simulink model "simulator_lqr_lpv"  (R2024a)
settings: Solver=FixedStepAuto  StartTime=0.0  StopTime=10  FixedStep=0.01  RelTol=1e-3
values from neighbouring files (symbols this model uses):
  ad = sys_d.A    [Project.m]
  bd = sys_d.B    [Project.m]
  BT_D = Ts * B_T    [Project.m]
  C_T = diag([1, 1, 1])    [Project.m]
  D_T = [0;0;0]    [Project.m]
  K1 = Y1*inv(P)    [Project.m]
  K2 = Y2*inv(P)    [Project.m]
  K3 = Y3*inv(P)    [Project.m]
  K4 = Y4*inv(P)    [Project.m]
  K_lqr = dlqr(ad, bd, Q_lqr, R_lqr)    [Project.m]
  Kk1 = Y1*inv(P)    [Project.m]
  Kk2 = Y2*inv(P)    [Project.m]
  Kk3 = Y3*inv(P)    [Project.m]
  rho1max = maxval    (= 20)    [Project.m]
  rho1min = minval    (= 5)    [Project.m]
  rho2max = 1/minval    (= 0.2)    [Project.m]
  rho2min = 1/maxval    (= 0.05)    [Project.m]
  Ts = 0.01    [Project.m]
  vx = 20    [Project.m]
libraries: cstblocks x2
settings Model: Creator=etudiant  LastModifiedBy=etudiant
settings DataIOCC: InspectSignalLogs=on

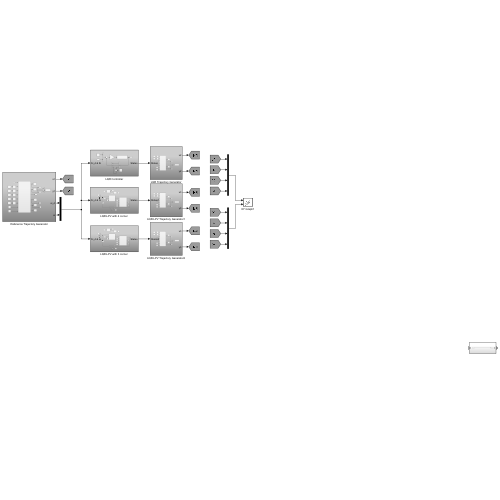
[thumbnail: Simulink's stored preview of the top-level diagram]
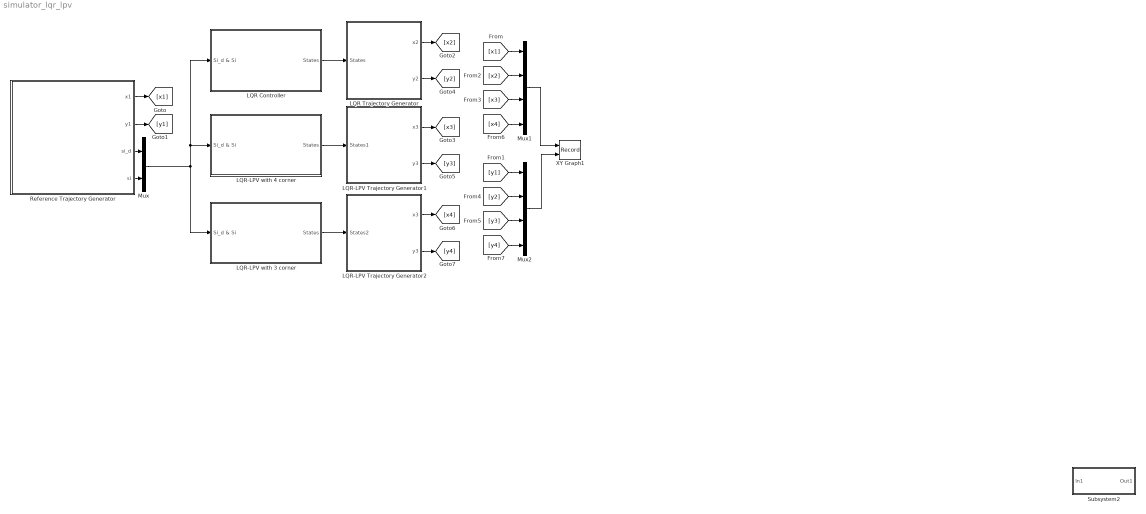
== system simulator_lqr_lpv ==
  LQR Controller : Subsystem
  LQR Trajectory Generator : Subsystem
  LQR-LPV Trajectory Generator1 : Subsystem
  LQR-LPV Trajectory Generator2 : Subsystem
  "LQR-LPV with 3 corner " : Subsystem
  "LQR-LPV with 4 corner " : Subsystem
  Mux : Mux  Inputs=2
  Mux1 : Mux
  Mux2 : Mux
  Reference Trajectory Generator : Subsystem
  Subsystem2 : Subsystem
  XY Graph1 : Record  FileSettingsInternal="{\"entries\":[{\"content\":{\"excelSettings\":{\"content\":{},\"type\":\"Streamout.ExcelSettings\"}},\"type\":\"Streamout.FileSettingStorage\",\"uuid\":\"\"}],\"packageUris\":[\"http:\\/\\/schema.mathworks.com\\/mf0\\/streamout_blocks\\/R2020a\"],\"version\":\"1.0\"}"  Layout=[1 1]  SignalsInternal="{\"entries\":[{\"content\":{\"signals\":[{\"content\":{\"blockPath\":[],\"dimensions\":[4],\"domain\":\"\",\"hasChildren\":true,\"lineColor\":\"#a2142f\",\"lineWidth\":2,\"port\":1,\"sid\":[\"\"],\"signalID\":1,\"signalName\":\"Mux1\"},\"type\":\"RecordBlkView.Signal\",\"uuid\":\"\"},{\"content\":{\"blockPath\":[],\"channel\":[1],\"dimensions\":[4],\"domain\":\"\",\"lineColor\":\"#fe330a\",\"lineWidth\":2,\"parentID\":1,\"plots\":[ 1 ],\"port\":1,\"sid\":[\"\"],\"signalID\":2,\"signalName\":\"Mux1\"},\"type\":\"RecordBlkView.Signal\",\"uuid\":\"\"},{\"content\":{\"blockPath\":[],\"dimensions\":[4],\"domain\":\"\",\"hasChildren\":true,\"lineColor\":\"#ff6929\",\"lineWidth\":2,\"port\":2,\"sid\":[\"\"],\"signalID\":3,\"signalName\":\"Mux2\"},\"type\":\"RecordBlkView.Signal\",\"uuid\":\"\"},{\"content\":{\"blockPath\":[],\"channel\":[1],\"dimensions\":[4],\"domain\":\"\",\"lineColor\":\"#fe330a\",\"lineWidth\":2,\"parentID\":3,\"plots\":[ 1 ],\"port\":2,\"sid\":[\"\"],\"signalID\":4,\"signalName\":\"Mux2\"},\"type\":\"RecordBlkView.Signal\",\"uuid\":\"\"},{\"content\":{\"blockPath\":[],\"channel\":[2],\"dimensions\":[4],\"domain\":\"\",\"lineColor\":\"#ff6929\",\"lineWidth\":2,\"parentID\":1,\"plots\":[ 1 ],\"port\":1,\"sid\":[\"\"],\"signalID\":5,\"signalName\":\"Mux1\"},\"type\":\"RecordBlkView.Signal\",\"uuid\":\"\"},{\"content\":{\"blockPath\":[],\"channel\":[3],\"dimensions\":[4],\"domain\":\"\",\"lineColor\":\"#b746ff\",\"lineWidth\":2,\"parentID\":1,\"plots\":[ 1 ],\"port\":1,\"sid\":[\"\"],\"signalID\":6,\"signalName\":\"Mux1\"},\"type\":\"RecordBlkView.Signal\",\"uuid\":\"\"},{\"content\":{\"blockPath\":[],\"channel\":[4],\"dimensions\":[4],\"domain\":\"\",\"lineColor\":\"#7e2f8e\",\"lineWidth\":2,\"parentID\":1,\"plots\":[ 1 ],\"port\":1,\"sid\":[\"\"],\"signalID\":7,\"signalName\":\"Mux1\"},\"type\":\"RecordBlkView.Signal\",\"uuid\":\"\"},{\"content\":{\"blockPath\":[],\"channel\":[2],\"dimensions\":[4],\"domain\":\"\",\"lineColor\":\"#64d413\",\"lineWidth\":2,\"parentID\":3,\"plots\":[ 1 ],\"port\":2,\"sid\":[\"\"],\"signalID\":8,\"signalName\":\"Mux2\"},\"type\":\"RecordBlkView.Signal\",\"uuid\":\"\"},{\"content\":{\"blockPath\":[],\"channel\":[3],\"dimensions\":[4],\"domain\":\"\",\"lineColor\":\"#ff13a6\",\"lineWidth\":2,\"parentID\":3,\"plots\":[ 1 ],\"port\":2,\"sid\":[\"\"],\"signalID\":9,\"signalName\":\"Mux2\"},\"type\":\"RecordBlkView.Signal\",\"uuid\":\"\"},{\"content\":{\"blockPath\":[],\"channel\":[4],\"dimensions\":[4],\"domain\":\"\",\"lineColor\":\"#a2142f\",\"lineWidth\":2,\"parentID\":3,\"plots\":[ 1 ],\"port\":2,\"sid\":[\"\"],\"signalID\":10,\"signalName\":\"Mux2\"},\"type\":\"RecordBlkView.Signal\",\"uuid\":\"\"}]},\"type\":\"RecordBlkView.InputSignals\",\"uuid\":\"\"}],\"packageUris\":[\"http:\\/\\/schema.mathworks.com\\/mf0\\/streamout_blocks\\/R2020a\"],\"version\":\"1.0\"}"  VisualizationBindings="{\"xyplotplugin\":{\"info\":[{\"series\":[{\"bindingParametersList\":[{\"parameter\":\"X-Axis\",\"signalID\":6,\"signalName\":\"Mux1(3)\"},{\"parameter\":\"Y-Axis\",\"signalID\":9,\"signalName\":\"Mux2(3)\"}],\"seriesID\":0},{\"bindingParametersList\":[{\"parameter\":\"X-Axis\",\"signalID\":2,\"signalName\":\"Mux1(1)\"},{\"parameter\":\"Y-Axis\",\"signalID\":4,\"signalName\":\"Mux2(1)\"}],\"seriesID\":1},{\"bindingParametersList\":[{\"parameter\":\"X-Axis\",\"signalID\":5,\"signalName\":\"Mux1(2)\"},{\"parameter\":\"Y-Axis\",\"signalID\":8,\"signalName\":\"Mux2(2)\"}],\"seriesID\":2},{\"bindingParametersList\":[{\"parameter\":\"X-Axis\",\"signalID\":7,\"signalName\":\"Mux1(4)\"},{\"parameter\":\"Y-Axis\",\"signalID\":10,\"signalName\":\"Mux2(4)\"}],\"seriesID\":3}],\"subplotID\":1}]}}"  CompatibilityTag=XY
  wires:
  LQR Controller/1(States) -> LQR Trajectory Generator/1(States)
  Reference Trajectory Generator/3(si_d) -> Mux/1
  Reference Trajectory Generator/4(si) -> Mux/2
  Mux1/1 -> XY Graph1/1
  Reference Trajectory Generator/1(x1) -> [x1]
  [x1] -> Mux1/1
  Reference Trajectory Generator/2(y1) -> [y1]
  [y1] -> Mux2/1
  LQR-LPV Trajectory Generator1/1(x3) -> [x3]
  LQR Trajectory Generator/1(x2) -> [x2]
  LQR-LPV Trajectory Generator1/2(y3) -> [y3]
  LQR Trajectory Generator/2(y2) -> [y2]
  [x3] -> Mux1/3
  [x2] -> Mux1/2
  Mux2/1 -> XY Graph1/2
  [y2] -> Mux2/2
  [y3] -> Mux2/3
  Mux/1 -> LQR Controller/1(Si_d & Si), "LQR-LPV with 4 corner "/1(Si_d & Si), "LQR-LPV with 3 corner "/1(Si_d & Si)
  "LQR-LPV with 4 corner "/1(States) -> LQR-LPV Trajectory Generator1/1(States1)
  "LQR-LPV with 3 corner "/1(States) -> LQR-LPV Trajectory Generator2/1(States2)
  LQR-LPV Trajectory Generator2/1(x3) -> [x4]
  LQR-LPV Trajectory Generator2/2(y3) -> [y4]
  [y4] -> Mux2/4
  [x4] -> Mux1/4

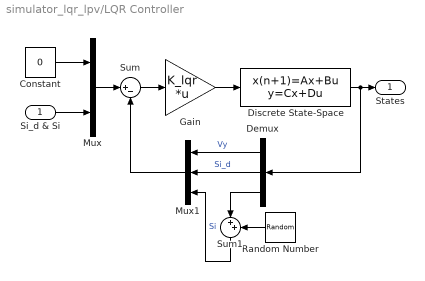
== system simulator_lqr_lpv/LQR Controller ==
  Si_d & Si : Inport
  Constant : Constant  Value=0  SampleTime=Ts
  Demux : Demux  Outputs=3
  Discrete State-Space : DiscreteStateSpace  A=ad  B=bd  C=eye(3)  D=[0;0;0];  SampleTime=Ts
  Gain : Gain  Gain=K_lqr  Multiplication=Matrix(K*u)
  Mux : Mux  Inputs=2
  Mux1 : Mux  Inputs=3
  Random Number : RandomNumber  Variance=15  SampleTime=0.1
  Sum : Sum  Inputs=|+-
  Sum1 : Sum  Inputs=|++
  States : Outport
  wires:
  Si_d & Si/1 -> Mux/2
  Gain/1 -> Discrete State-Space/1
  Sum/1 -> Gain/1
  Mux/1 -> Sum/1
  Constant/1 -> Mux/1
  Mux1/1 -> Sum/2
  Demux/2 -> Mux1/2  "Si_d"
  Demux/1 -> Mux1/1  "Vy"
  Discrete State-Space/1 -> Demux/1, States/1
  Demux/3 -> Sum1/1
  Random Number/1 -> Sum1/2
  Sum1/1 -> Mux1/3  "Si"

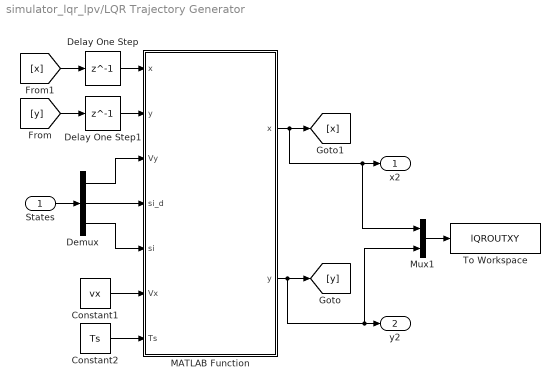
== system simulator_lqr_lpv/LQR Trajectory Generator ==
  States : Inport
  Constant1 : Constant  Value=vx  SampleTime=Ts
  Constant2 : Constant  Value=Ts  SampleTime=Ts
  Delay One Step : Delay  DelayLength=1
  Delay One Step1 : Delay  DelayLength=1
  Demux : Demux  Outputs=3
  MATLAB Function : MATLAB Function  TreatAsAtomicUnit=on
  Mux1 : Mux  Inputs=2
  To Workspace : ToWorkspace  VariableName=lQROUTXY  SampleTime=Ts
  x2 : Outport
  y2 : Outport  Port=2
  wires:
  Demux/3 -> MATLAB Function/5(si)
  Delay One Step/1 -> MATLAB Function/1("x ")
  Demux/2 -> MATLAB Function/4(si_d)
  Delay One Step1/1 -> MATLAB Function/2("y ")
  Constant2/1 -> MATLAB Function/7(Ts)
  Demux/1 -> MATLAB Function/3(Vy)
  Mux1/1 -> To Workspace/1
  Constant1/1 -> MATLAB Function/6(Vx)
  States/1 -> Demux/1
  [y] -> Delay One Step1/1
  [x] -> Delay One Step/1
  MATLAB Function/1(x) -> Mux1/1, x2/1, [x]
  MATLAB Function/2(y) -> [y], Mux1/2, y2/1

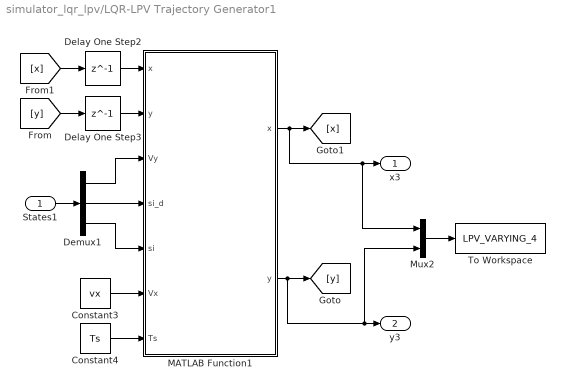
== system simulator_lqr_lpv/LQR-LPV Trajectory Generator1 ==
  States1 : Inport
  Constant3 : Constant  Value=vx  SampleTime=Ts
  Constant4 : Constant  Value=Ts  SampleTime=Ts
  Delay One Step2 : Delay  DelayLength=1
  Delay One Step3 : Delay  DelayLength=1
  Demux1 : Demux  Outputs=3
  MATLAB Function1 : MATLAB Function  TreatAsAtomicUnit=on
  Mux2 : Mux  Inputs=2
  To Workspace : ToWorkspace  VariableName=LPV_VARYING_4  SampleTime=Ts
  x3 : Outport
  y3 : Outport  Port=2
  wires:
  [y] -> Delay One Step3/1
  MATLAB Function1/2(y) -> [y], Mux2/2, y3/1
  [x] -> Delay One Step2/1
  MATLAB Function1/1(x) -> Mux2/1, x3/1, [x]
  Delay One Step2/1 -> MATLAB Function1/1("x ")
  Demux1/1 -> MATLAB Function1/3(Vy)
  Mux2/1 -> To Workspace/1
  Constant4/1 -> MATLAB Function1/7(Ts)
  States1/1 -> Demux1/1
  Delay One Step3/1 -> MATLAB Function1/2("y ")
  Constant3/1 -> MATLAB Function1/6(Vx)
  Demux1/2 -> MATLAB Function1/4(si_d)
  Demux1/3 -> MATLAB Function1/5(si)

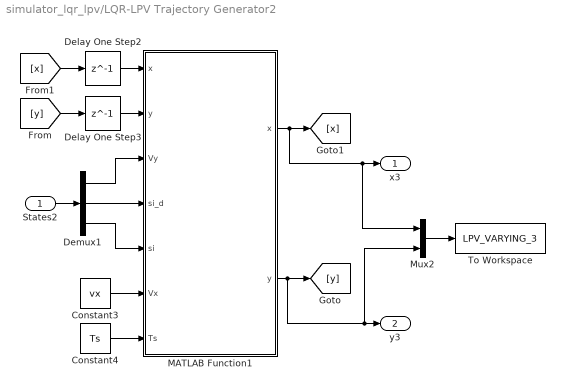
== system simulator_lqr_lpv/LQR-LPV Trajectory Generator2 ==
  States2 : Inport
  Constant3 : Constant  Value=vx  SampleTime=Ts
  Constant4 : Constant  Value=Ts  SampleTime=Ts
  Delay One Step2 : Delay  DelayLength=1
  Delay One Step3 : Delay  DelayLength=1
  Demux1 : Demux  Outputs=3
  MATLAB Function1 : MATLAB Function  TreatAsAtomicUnit=on
  Mux2 : Mux  Inputs=2
  To Workspace : ToWorkspace  VariableName=LPV_VARYING_3  SampleTime=Ts
  x3 : Outport
  y3 : Outport  Port=2
  wires:
  [y] -> Delay One Step3/1
  MATLAB Function1/2(y) -> [y], Mux2/2, y3/1
  [x] -> Delay One Step2/1
  MATLAB Function1/1(x) -> Mux2/1, x3/1, [x]
  Delay One Step2/1 -> MATLAB Function1/1("x ")
  Demux1/1 -> MATLAB Function1/3(Vy)
  Mux2/1 -> To Workspace/1
  Constant4/1 -> MATLAB Function1/7(Ts)
  States2/1 -> Demux1/1
  Delay One Step3/1 -> MATLAB Function1/2("y ")
  Constant3/1 -> MATLAB Function1/6(Vx)
  Demux1/2 -> MATLAB Function1/4(si_d)
  Demux1/3 -> MATLAB Function1/5(si)

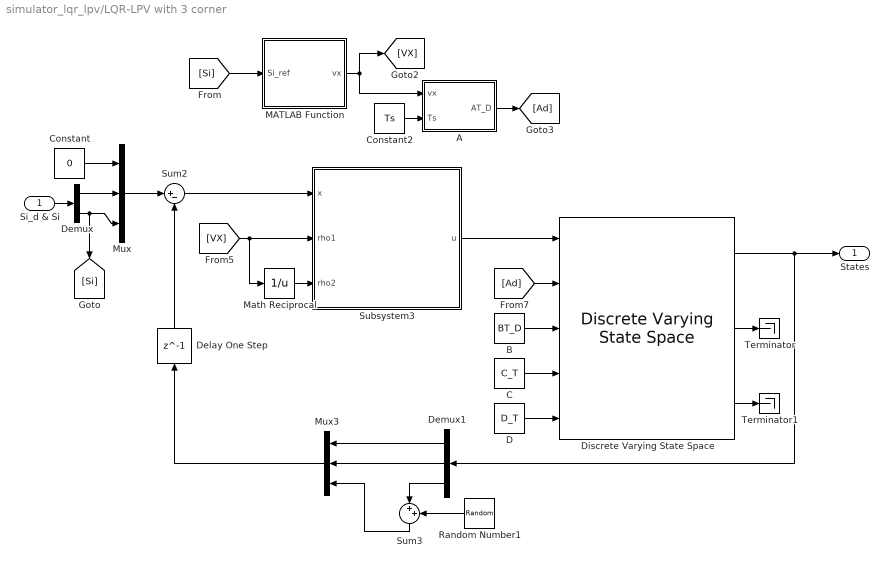
== system simulator_lqr_lpv/LQR-LPV with 3 corner  ==
  Si_d & Si : Inport
  A : MATLAB Function  TreatAsAtomicUnit=on
  B : Constant  Value=BT_D  SampleTime=Ts
  C : Constant  Value=C_T  SampleTime=Ts
  Constant : Constant  Value=0  SampleTime=Ts
  Constant2 : Constant  Value=Ts  SampleTime=Ts
  D : Constant  Value=D_T  SampleTime=Ts
  Delay One Step : Delay  DelayLength=1
  Demux : Demux  Outputs=2
  Demux1 : Demux  Outputs=3
  Discrete Varying State Space : cstblocks/Linear Parameter Varying/Discrete Varying State Space  x0=0  Ts=-1  OutputX=on  OutputDX=on  Feedthrough=on  InputX0=off  InputDX0=off  InputU0=off  InputY0=off
  MATLAB Function : MATLAB Function  TreatAsAtomicUnit=on
  Math Reciprocal : Math  Operator=reciprocal  SignedPower=on
  Mux : Mux  Inputs=3
  Mux3 : Mux  Inputs=3
  Random Number1 : RandomNumber  Variance=15  SampleTime=Ts
  Subsystem3 : Subsystem
  Sum2 : Sum  Inputs=|+-
  Sum3 : Sum  Inputs=|++
  Terminator : Terminator
  Terminator1 : Terminator
  States : Outport
  wires:
  Constant/1 -> Mux/1
  Demux1/2 -> Mux3/2
  Sum3/1 -> Mux3/3
  C/1 -> Discrete Varying State Space/4
  D/1 -> Discrete Varying State Space/5
  [Ad] -> Discrete Varying State Space/2
  [VX] -> Math Reciprocal/1, Subsystem3/2(rho1)
  Discrete Varying State Space/3 -> Terminator1/1
  Discrete Varying State Space/1 -> States/1, Demux1/1
  Discrete Varying State Space/2 -> Terminator/1
  Demux1/1 -> Mux3/1
  Sum2/1 -> Subsystem3/1(x)
  Subsystem3/1("u ") -> Discrete Varying State Space/1
  Mux/1 -> Sum2/1
  Constant2/1 -> A/2(Ts)
  MATLAB Function/1(vx) -> [VX], A/1(vx)
  A/1(AT_D) -> [Ad]
  Si_d & Si/1 -> Demux/1
  Demux/1 -> Mux/2
  Demux/2 -> [Si], Mux/3
  [Si] -> MATLAB Function/1(Si_ref)
  Mux3/1 -> Delay One Step/1
  Random Number1/1 -> Sum3/2
  Demux1/3 -> Sum3/1
  B/1 -> Discrete Varying State Space/3
  Math Reciprocal/1 -> Subsystem3/3(rho2)
  Delay One Step/1 -> Sum2/2

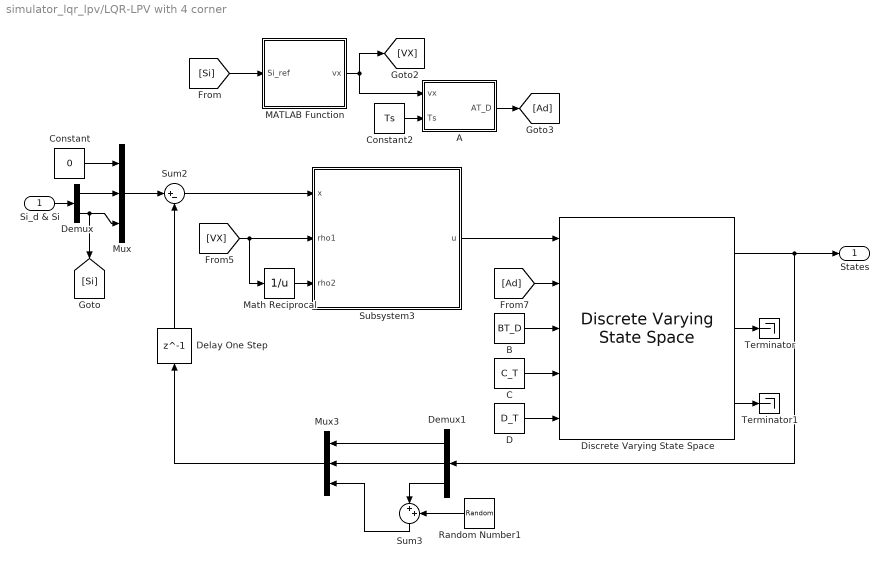
== system simulator_lqr_lpv/LQR-LPV with 4 corner  ==
  Si_d & Si : Inport
  A : MATLAB Function  TreatAsAtomicUnit=on
  B : Constant  Value=BT_D  SampleTime=Ts
  C : Constant  Value=C_T  SampleTime=Ts
  Constant : Constant  Value=0  SampleTime=Ts
  Constant2 : Constant  Value=Ts  SampleTime=Ts
  D : Constant  Value=D_T  SampleTime=Ts
  Delay One Step : Delay  DelayLength=1
  Demux : Demux  Outputs=2
  Demux1 : Demux  Outputs=3
  Discrete Varying State Space : cstblocks/Linear Parameter Varying/Discrete Varying State Space  x0=0  Ts=-1  OutputX=on  OutputDX=on  Feedthrough=on  InputX0=off  InputDX0=off  InputU0=off  InputY0=off
  MATLAB Function : MATLAB Function  TreatAsAtomicUnit=on
  Math Reciprocal : Math  Operator=reciprocal  SignedPower=on
  Mux : Mux  Inputs=3
  Mux3 : Mux  Inputs=3
  Random Number1 : RandomNumber  Variance=15  SampleTime=Ts
  Subsystem3 : Subsystem
  Sum2 : Sum  Inputs=|+-
  Sum3 : Sum  Inputs=|++
  Terminator : Terminator
  Terminator1 : Terminator
  States : Outport
  wires:
  Constant/1 -> Mux/1
  Demux1/2 -> Mux3/2
  Sum3/1 -> Mux3/3
  C/1 -> Discrete Varying State Space/4
  D/1 -> Discrete Varying State Space/5
  [Ad] -> Discrete Varying State Space/2
  [VX] -> Math Reciprocal/1, Subsystem3/2(rho1)
  Discrete Varying State Space/3 -> Terminator1/1
  Discrete Varying State Space/1 -> States/1, Demux1/1
  Discrete Varying State Space/2 -> Terminator/1
  Demux1/1 -> Mux3/1
  Sum2/1 -> Subsystem3/1(x)
  Subsystem3/1("u ") -> Discrete Varying State Space/1
  Mux/1 -> Sum2/1
  Constant2/1 -> A/2(Ts)
  MATLAB Function/1(vx) -> [VX], A/1(vx)
  A/1(AT_D) -> [Ad]
  Si_d & Si/1 -> Demux/1
  Demux/1 -> Mux/2
  Demux/2 -> [Si], Mux/3
  [Si] -> MATLAB Function/1(Si_ref)
  Mux3/1 -> Delay One Step/1
  Random Number1/1 -> Sum3/2
  Demux1/3 -> Sum3/1
  B/1 -> Discrete Varying State Space/3
  Math Reciprocal/1 -> Subsystem3/3(rho2)
  Delay One Step/1 -> Sum2/2

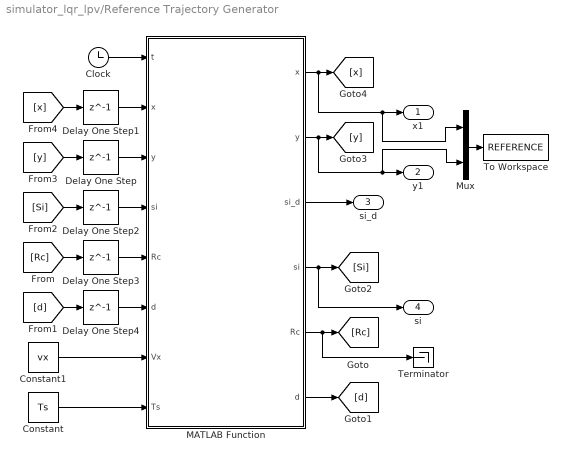
== system simulator_lqr_lpv/Reference Trajectory Generator ==
  Clock : Clock
  Constant : Constant  Value=Ts  SampleTime=Ts
  Constant1 : Constant  Value=vx  SampleTime=Ts
  Delay One Step{,1..4} (5 alike) : Delay  DelayLength=1
  MATLAB Function : MATLAB Function  TreatAsAtomicUnit=on
  Mux : Mux  Inputs=2
  Terminator : Terminator
  To Workspace : ToWorkspace  VariableName=REFERENCE  SampleTime=Ts
      settings: Save2DSignal=2-D array (concatenate along first dimension)
  x1 : Outport
  y1 : Outport  Port=2
  si_d : Outport  Port=3
  si : Outport  Port=4
  wires:
  Delay One Step1/1 -> MATLAB Function/2("x ")
  Clock/1 -> MATLAB Function/1(t)
  Delay One Step4/1 -> MATLAB Function/6("d ")
  Delay One Step/1 -> MATLAB Function/3("y ")
  Delay One Step3/1 -> MATLAB Function/5("Rc ")
  Delay One Step2/1 -> MATLAB Function/4("si ")
  Constant/1 -> MATLAB Function/8(Ts)
  Constant1/1 -> MATLAB Function/7(Vx)
  MATLAB Function/3(si_d) -> si_d/1
  MATLAB Function/5(Rc) -> Terminator/1, [Rc]
  [Rc] -> Delay One Step3/1
  MATLAB Function/6(d) -> [d]
  [d] -> Delay One Step4/1
  [Si] -> Delay One Step2/1
  MATLAB Function/4(si) -> si/1, [Si]
  MATLAB Function/2(y) -> y1/1, Mux/2, [y]
  [y] -> Delay One Step/1
  MATLAB Function/1(x) -> x1/1, Mux/1, [x]
  [x] -> Delay One Step1/1
  Mux/1 -> To Workspace/1

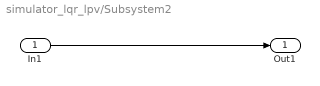
== system simulator_lqr_lpv/Subsystem2 ==
  In1 : Inport
  Out1 : Outport
  wires:
  In1/1 -> Out1/1

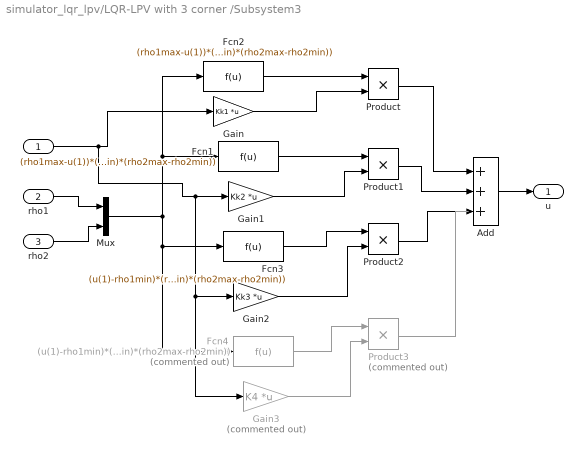
== system simulator_lqr_lpv/LQR-LPV with 3 corner /Subsystem3 ==
  x : Inport
  rho1 : Inport  Port=2
  rho2 : Inport  Port=3
  Add : Sum  Inputs=+++
  Fcn1 : Fcn  Expr=(rho1max-u(1))*(u(2)-rho2min)/((rho1max-rho1min)*(rho2max-rho2min))
  Fcn2 : Fcn  Expr=(rho1max-u(1))*(rho2max-u(2))/((rho1max-rho1min)*(rho2max-rho2min))
  Fcn3 : Fcn  Expr=(u(1)-rho1min)*(rho2max-u(2))/((rho1max-rho1min)*(rho2max-rho2min))
  Fcn4 : Fcn  Commented=on  Expr=(u(1)-rho1min)*(u(2)-rho2min)/((rho1max-rho1min)*(rho2max-rho2min))
  Gain : Gain  Gain=Kk1  Multiplication=Matrix(K*u)
  Gain1 : Gain  Gain=Kk2  Multiplication=Matrix(K*u)
  Gain2 : Gain  Gain=Kk3  Multiplication=Matrix(K*u)
  Gain3 : Gain  Commented=on  Gain=K4  Multiplication=Matrix(K*u)
  Mux : Mux  Inputs=2
  Product : Product
  Product1 : Product
  Product2 : Product
  Product3 : Product  Commented=on
  "u " : Outport  VectorParamsAs1DForOutWhenUnconnected=off
  wires:
  Fcn2/1 -> Product/1
  Gain/1 -> Product/2
  Product/1 -> Add/1
  Product1/1 -> Add/2
  Gain1/1 -> Product1/2
  Fcn1/1 -> Product1/1
  Add/1 -> "u "/1
  rho1/1 -> Mux/1
  rho2/1 -> Mux/2
  Mux/1 -> Fcn1/1, Fcn2/1, Fcn4/1, Fcn3/1
  Product2/1 -> Add/3
  Product3/1 -> ?
  Fcn4/1 -> Product3/1
  Gain3/1 -> Product3/2
  Fcn3/1 -> Product2/1
  Gain2/1 -> Product2/2
  x/1 -> Gain2/1, Gain3/1, Gain1/1, Gain/1

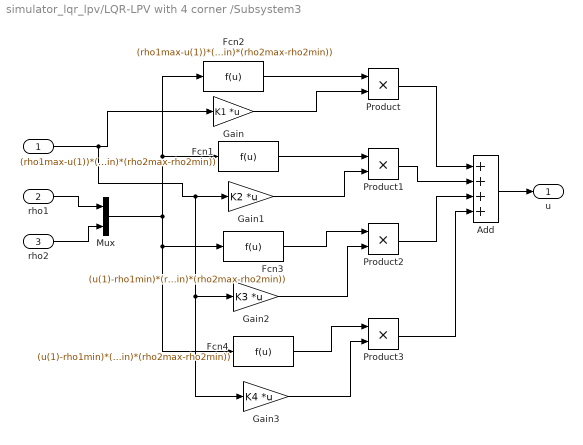
== system simulator_lqr_lpv/LQR-LPV with 4 corner /Subsystem3 ==
  x : Inport
  rho1 : Inport  Port=2
  rho2 : Inport  Port=3
  Add : Sum  Inputs=++++
  Fcn1 : Fcn  Expr=(rho1max-u(1))*(u(2)-rho2min)/((rho1max-rho1min)*(rho2max-rho2min))
  Fcn2 : Fcn  Expr=(rho1max-u(1))*(rho2max-u(2))/((rho1max-rho1min)*(rho2max-rho2min))
  Fcn3 : Fcn  Expr=(u(1)-rho1min)*(rho2max-u(2))/((rho1max-rho1min)*(rho2max-rho2min))
  Fcn4 : Fcn  Expr=(u(1)-rho1min)*(u(2)-rho2min)/((rho1max-rho1min)*(rho2max-rho2min))
  Gain : Gain  Gain=K1  Multiplication=Matrix(K*u)
  Gain1 : Gain  Gain=K2  Multiplication=Matrix(K*u)
  Gain2 : Gain  Gain=K3  Multiplication=Matrix(K*u)
  Gain3 : Gain  Gain=K4  Multiplication=Matrix(K*u)
  Mux : Mux  Inputs=2
  Product{,1..3} (4 alike) : Product
  "u " : Outport  VectorParamsAs1DForOutWhenUnconnected=off
  wires:
  Fcn2/1 -> Product/1
  Gain/1 -> Product/2
  Product/1 -> Add/1
  Product1/1 -> Add/2
  Gain1/1 -> Product1/2
  Fcn1/1 -> Product1/1
  Add/1 -> "u "/1
  rho1/1 -> Mux/1
  rho2/1 -> Mux/2
  Mux/1 -> Fcn1/1, Fcn2/1, Fcn4/1, Fcn3/1
  Product2/1 -> Add/3
  Product3/1 -> Add/4
  Fcn4/1 -> Product3/1
  Gain3/1 -> Product3/2
  Fcn3/1 -> Product2/1
  Gain2/1 -> Product2/2
  x/1 -> Gain2/1, Gain3/1, Gain1/1, Gain/1

== matlab function simulator_lqr_lpv/LQR Trajectory Generator/MATLAB Function ==
  data: x output; x input; y output; y input; Vy input; si_d input; si input; Vx input; Ts input
function [x, y]  = lqr_trajectory(x, y,  Vy, si_d,si,Vx,Ts)

si=si+si_d*Ts;
x=x +Vx*Ts*cos(si)+ Vy*Ts*sin(si);
y=y +Vx*Ts*sin(si)+Vy*Ts*cos(si);

end

== matlab function simulator_lqr_lpv/Reference Trajectory Generator/MATLAB Function ==
  data: x output; t input; y output; si_d output; x input; y input; si input; Rc input; d input; Vx input; Ts input; si output; Rc output; d output
function [x, y,si_d,si, Rc, d]  = Desired_Trajectory(t,x, y, si, Rc,  d, Vx, Ts)
t=t+1;

Vy=0;
RD=100;

d=d+Vx*Ts;
    if d<40 
       Rc=0;
    elseif d<80
        Rc=Rc+Ts*(1/RD);
    else
        Rc=Rc;
    end
si=si+Rc*Vx*Ts;
si_d=Rc*Vx;
x=x +Vx*Ts*cos(si);
y=y +Vx*Ts*sin(si);

== matlab function simulator_lqr_lpv/LQR-LPV with 3 corner /A ==
  data: vx input; AT_D output; Ts input
function AT_D= fcn(vx,Ts)

   Cf = 57117; %N*rad^-1
Cr = 81396; %N*rad^-1
Iz = 1975; %kg*m^2
m = 1621; %Kg
g = 9.8; %m/s^2
Lf = 1.15; %m
Lr = 0.20; %m wheel radius

    A_T= [-(Cf + Cr)/(m*vx) ,-vx+ (Cr*Lr - Cf*Lf)/(m*vx), 0;
         (-Lf*Cf + Lr*Cr)/(Iz*vx), -(Lf^2*Cf + Lr^2*Cr)/(Iz*vx),  0;
         0, 1, 0];
    AT_D=eye(size(A_T))+Ts*A_T;

end

== matlab function simulator_lqr_lpv/LQR-LPV with 4 corner /MATLAB Function ==
  data: Si_ref input; vx output
function vx  = velocity_in_x(Si_ref)
            % Default value for Vx
           vx =10;
        if Si_ref==0
            vx=17;
        end 
        if Si_ref>1
            vx=30;
        end
        if Si_ref>=1
            vx=7;
        end 
        if Si_ref>=1.6
            vx=8;
        end 
end

== matlab function simulator_lqr_lpv/LQR-LPV with 4 corner /A ==
  data: vx input; AT_D output; Ts input
function AT_D= fcn(vx,Ts)

   Cf = 57117; %N*rad^-1
Cr = 81396; %N*rad^-1
Iz = 1975; %kg*m^2
m = 1621; %Kg
g = 9.8; %m/s^2
Lf = 1.15; %m
Lr = 0.20; %m wheel radius

    A_T= [-(Cf + Cr)/(m*vx) ,-vx+ (Cr*Lr - Cf*Lf)/(m*vx), 0;
         (-Lf*Cf + Lr*Cr)/(Iz*vx), -(Lf^2*Cf + Lr^2*Cr)/(Iz*vx),  0;
         0, 1, 0];
    AT_D=eye(size(A_T))+Ts*A_T;

end

== matlab function simulator_lqr_lpv/LQR-LPV with 3 corner /MATLAB Function ==
  data: Si_ref input; vx output
function vx  = velocity_in_x(Si_ref)
            % Default value for Vx
           vx =10;
        if Si_ref==0
            vx=17;
        end 
        if Si_ref>1
            vx=30;
        end
        if Si_ref>=1
            vx=7;
        end 
        if Si_ref>=1.6
            vx=8;
        end 
end

== matlab function simulator_lqr_lpv/LQR-LPV Trajectory Generator1/MATLAB Function1 ==
  data: x output; x input; y output; y input; Vy input; si_d input; si input; Vx input; Ts input
function [x, y]  = lqr_lpv_trajectory(x, y,  Vy, si_d,si,Vx,Ts)

si=si+si_d*Ts;
x=x +Vx*Ts*cos(si)+ Vy*Ts*sin(si);
y=y +Vx*Ts*sin(si)+Vy*Ts*cos(si);
end

== matlab function simulator_lqr_lpv/LQR-LPV Trajectory Generator2/MATLAB Function1 ==
  data: x output; x input; y output; y input; Vy input; si_d input; si input; Vx input; Ts input
function [x, y]  = lqr_lpv_trajectory(x, y,  Vy, si_d,si,Vx,Ts)

si=si+si_d*Ts;
x=x +Vx*Ts*cos(si)+ Vy*Ts*sin(si);
y=y +Vx*Ts*sin(si)+Vy*Ts*cos(si);
end
